simulink model "practice_example"  (R2020a)
settings: Solver=VariableStepAuto  StartTime=0.0  StopTime=10.0  RelTol=1e-3
settings Model: Creator=Ganesh  LastModifiedBy=Ganesh

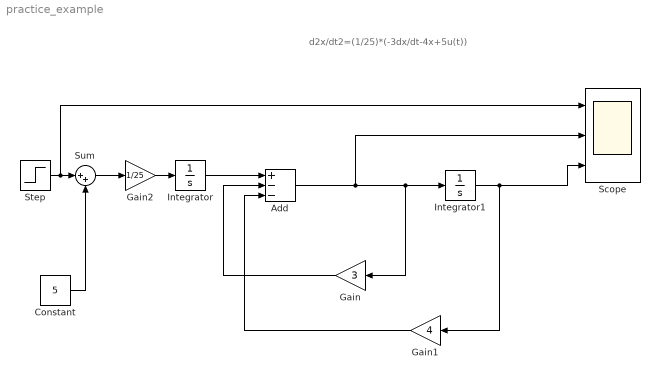
== system practice_example ==
  note: d2x/dt2=(1/25)*(-3dx/dt-4x+5u(t))
  Add : Sum  Inputs=+--
  Constant : Constant  Value=5
  Gain : Gain  Gain=3
  Gain1 : Gain  Gain=4
  Gain2 : Gain  Gain=1/25
  Integrator : Integrator
  Integrator1 : Integrator
  Scope : Scope  NumInputPorts=3
  Step : Step  SampleTime=0
  Sum : Sum  Inputs=|++
  wires:
  Integrator/1 -> Add/1
  Gain/1 -> Add/2
  Gain1/1 -> Add/3
  Add/1 -> Scope/2, Gain/1, Integrator1/1
  Integrator1/1 -> Scope/3, Gain1/1
  Constant/1 -> Sum/2
  Gain2/1 -> Integrator/1
  Sum/1 -> Gain2/1
  Step/1 -> Scope/1, Sum/1
